simulink model "punto5_daBaA"  (R2023a)
settings: Solver=VariableStepAuto  StartTime=0.0  StopTime=2000  RelTol=1e-3
values from neighbouring files (symbols this model uses):
  Pn1 = 100e6    (= 100000000)    [punto5_codice.m]
  Pn2 = 50e6    (= 50000000)    [punto5_codice.m]
  tau1 = 10    [punto5_codice.m]
  tau2 = 5    [punto5_codice.m]
libraries: simulink x2
settings Model: Creator=Samsung  LastModifiedBy=Samsung

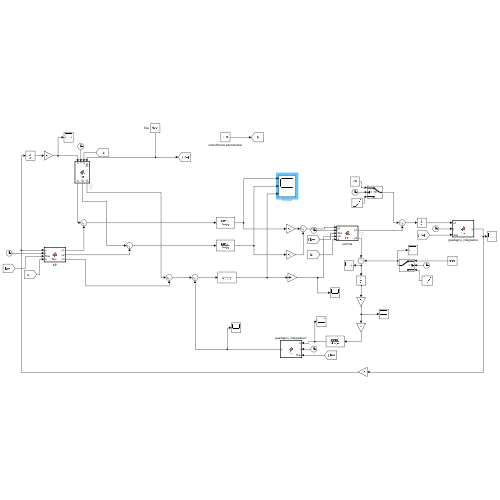
[thumbnail: Simulink's stored preview of the top-level diagram]
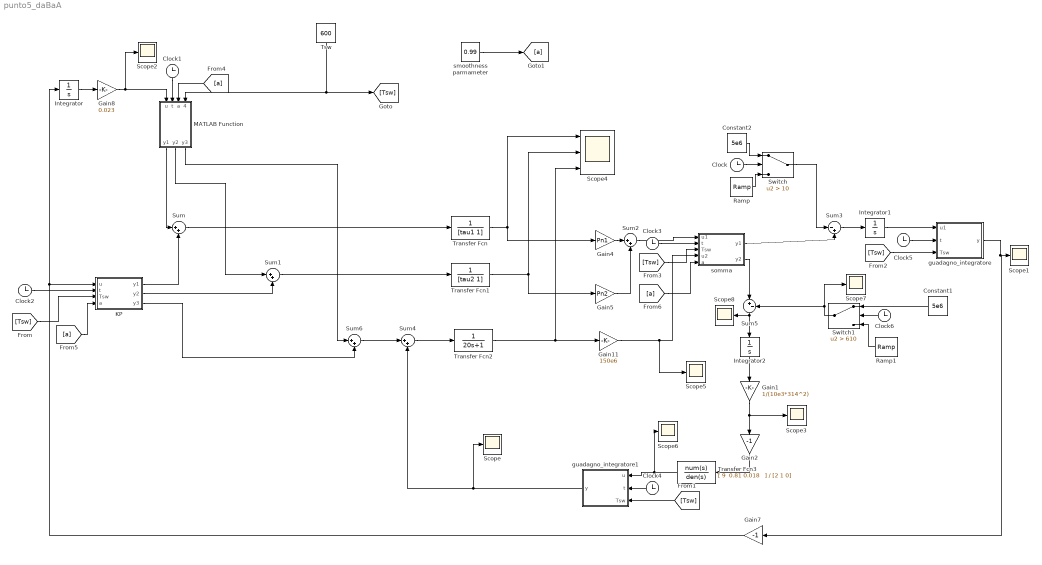
== system punto5_daBaA ==
  Clock{,1..6} (7 alike) : Clock
  Constant1 : Constant  Value=5e6
  Constant2 : Constant  Value=5e6
  Gain1 : Gain  Gain=1/(10e3*314^2)
  Gain11 : Gain  Gain=150e6
  Gain2 : Gain  Gain=-1
  Gain4 : Gain  Gain=Pn1
  Gain5 : Gain  Gain=Pn2
  Gain7 : Gain  Gain=-1
  Gain8 : Gain  Gain=0.023
  Integrator : Integrator
  Integrator1 : Integrator
  Integrator2 : Integrator
  KP : MATLAB Function  TreatAsAtomicUnit=on
  MATLAB Function : MATLAB Function  TreatAsAtomicUnit=on
  Ramp : simulink/Sources/Ramp  slope=500000  start=0  InitialOutput=0
  Ramp1 : simulink/Sources/Ramp  slope=500000  start=600  InitialOutput=0
  Scope{,1..3,5..8} (8 alike) : Scope
  Scope4 : Scope  NumInputPorts=3
  Sum{,1..2,4,6} (5 alike) : Sum  Inputs=|++
  Sum3 : Sum  Inputs=|-+
  Sum5 : Sum  Inputs=|+-
  Switch : Switch  Criteria=u2 > Threshold  Threshold=10  SaturateOnIntegerOverflow=off  InputSameDT=off
  Switch1 : Switch  Criteria=u2 > Threshold  Threshold=610  SaturateOnIntegerOverflow=off  InputSameDT=off
  Transfer Fcn : TransferFcn  Denominator=[tau1 1]
  Transfer Fcn1 : TransferFcn  Denominator=[tau2 1]
  Transfer Fcn2 : TransferFcn  Denominator=[20 1]
  Transfer Fcn3 : TransferFcn  Numerator="[ 9  0.81 0.018   ]"  Denominator=[2 1 0]
  Tsw : Constant  Value=600
  guadagno_integratore : MATLAB Function  TreatAsAtomicUnit=on
  guadagno_integratore1 : MATLAB Function  TreatAsAtomicUnit=on
  smoothness parmameter : Constant  Value=0.99
  somma : MATLAB Function  TreatAsAtomicUnit=on
  wires:
  [a] -> KP/4(a)
  [a] -> MATLAB Function/3(a)
  Switch/1 -> Sum3/1
  smoothness parmameter/1 -> [a]
  [Tsw] -> guadagno_integratore1/3(Tsw)
  [Tsw] -> KP/3(Tsw)
  Tsw/1 -> [Tsw], MATLAB Function/4(Tsw)
  somma/1(y1) -> Sum3/2
  MATLAB Function/3(y3) -> Sum6/1
  KP/1(y1) -> Sum/2
  MATLAB Function/1(y1) -> Sum/1
  Clock/1 -> Switch/2
  Sum5/1 -> Integrator2/1, Scope8/1
  somma/2(y2) -> Sum5/1
  Gain8/1 -> Scope2/1, MATLAB Function/1(u)
  Transfer Fcn2/1 -> Gain11/1, Scope4/3
  guadagno_integratore/1(y) -> Scope1/1, Gain7/1
  Gain7/1 -> Integrator/1, KP/1(u)
  Sum/1 -> Transfer Fcn/1
  MATLAB Function/2(y2) -> Sum1/1
  Gain5/1 -> Sum2/2
  Clock5/1 -> guadagno_integratore/2(t)
  Clock6/1 -> Switch1/2
  Sum6/1 -> Sum4/1
  guadagno_integratore1/1(y) -> Scope/1, Sum4/2
  Constant2/1 -> Switch/1
  Clock1/1 -> MATLAB Function/2(t)
  Sum4/1 -> Transfer Fcn2/1
  Transfer Fcn3/1 -> Scope6/1, guadagno_integratore1/1(u)
  Integrator/1 -> Gain8/1
  Switch1/1 -> Sum5/2, Scope7/1
  Gain1/1 -> Scope3/1, Gain2/1
  Gain11/1 -> Scope5/1, somma/4(u2)
  [Tsw] -> guadagno_integratore/3(Tsw)
  Integrator1/1 -> guadagno_integratore/1(u1)
  Integrator2/1 -> Gain1/1
  Transfer Fcn1/1 -> Gain5/1, Scope4/2
  Gain4/1 -> Sum2/1
  Clock4/1 -> guadagno_integratore1/2(t)
  KP/3(y3) -> Sum6/2
  Ramp/1 -> Switch/3
  Clock2/1 -> KP/2(t)
  KP/2(y2) -> Sum1/2
  Sum3/1 -> Integrator1/1
  Gain2/1 -> Transfer Fcn3/1
  Sum1/1 -> Transfer Fcn1/1
  Sum2/1 -> somma/1(u1)
  [Tsw] -> somma/3(Tsw)
  Clock3/1 -> somma/2(t)
  Transfer Fcn/1 -> Gain4/1, Scope4/1
  Constant1/1 -> Switch1/1
  [a] -> somma/5(a)
  Ramp1/1 -> Switch1/3

== matlab function punto5_daBaA/KP ==
  data: u input; y1 output; t input; y2 output; y3 output; Tsw input; a input
function [y1, y2,y3] = fcn(u, t, Tsw, a)
if t<Tsw
    y1=0.91*u;   
    y2=4.773*u;
    y3=0.182*u;
else 
    y1=(0.014*(1-a^(t-Tsw))+0.91*a^(t-Tsw))*u;
    y2=(3.686*(1-a^(t-Tsw))+4.773*a^(t-Tsw))*u;
    y3=0.182*a^(t-Tsw)*u;
end

== matlab function punto5_daBaA/MATLAB Function ==
  data: u input; y1 output; t input; a input; y2 output; y3 output; Tsw input
function [y1,y2,y3] = fcn(u, t, a, Tsw)
 if t<Tsw
    y3=0.4*u;
    y2=0.2*u;
    y1=0.4*u;
  else 
    y1=(1/3*(1-a^(t-Tsw))+0.4*a^(t-Tsw))*u;
    y2=(2/3*(1-a^(t-Tsw))+0.2*a^(t-Tsw))*u;
    y3=0.4*a^(t-Tsw)*u;
 
end

== matlab function punto5_daBaA/somma ==
  data: u1 input; t input; Tsw input; u2 input; y1 output; y2 output; a input
function [y1, y2] = fcn(u1, t, Tsw, u2, a)
if t<Tsw
    y1=(u1+u2); 
    y2=0;
else 
    y1=u1; 
    y2=u2;
end

== matlab function punto5_daBaA/guadagno_integratore ==
  data: u1 input; y output; t input; Tsw input
function y = fcn(u1, t, Tsw)
if t<Tsw
    y=1/(40e3*314^2)*u1;
else 
    y=1/(30e3*314^2)*u1; 
end

== matlab function punto5_daBaA/guadagno_integratore1 ==
  data: u input; y output; t input; Tsw input
function y = fcn(u,t, Tsw)
if t<Tsw
    y=0;
else 
    y=u; 
end
